simulink model "galvoMdl"  (R2015a)
settings: Solver=ode45  StartTime=0.0  StopTime=10.0  RelTol=1e-3
values from neighbouring files (symbols this model uses):
  JR = 7.3E-9    [dataDict_galvoLSK040EF.sldd]    (also in dataDict_galvoMod6860.sldd = 6.0E-8
  KEL = 0.015    [dataDict_galvoLSK040EF.sldd]    (also in dataDict_galvoMod6860.sldd = 0.0093
  KFR = 4.0E-6    [dataDict_galvoLSK040EF.sldd]    (also in dataDict_galvoMod6860.sldd = 1.0E-10
  L = 0.0018    [dataDict_galvoLSK040EF.sldd]    (also in dataDict_galvoMod6860.sldd = 0.00016
  RL = 2.3    [dataDict_galvoLSK040EF.sldd]    (also in dataDict_galvoMod6860.sldd = 1.5
undefined symbols (not defined in the file or in its folder): KME
settings Model: Creator=mainster  LastModifiedBy=mainster
settings DebuggingCC: UnderspecifiedInitializationDetection=Classic  MergeDetectMultiDrivingBlocksExec=none  SolverPrmCheckMsg=warning  StateNameClashWarn=warning

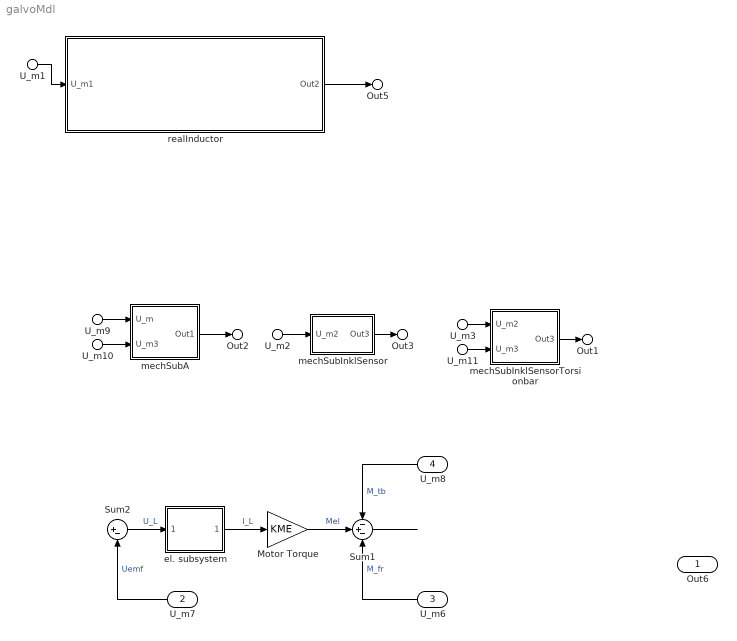
== system galvoMdl ==
  U_m1 : Inport
  U_m7 : Inport  Port=2
  U_m6 : Inport  Port=3
  U_m8 : Inport  Port=4
  U_m9 : Inport  Port=5
  U_m10 : Inport  Port=6
  U_m2 : Inport  Port=7
  U_m3 : Inport  Port=8
  U_m11 : Inport  Port=9
  Motor Torque : Gain  Gain=KME
  Sum1 : Sum  Inputs=-+-
  Sum2 : Sum  Inputs=|+-
  el. subsystem : Subsystem
  mechSubA : Subsystem
  mechSubInklSensor : Subsystem
  mechSubInklSensorTorsionbar : Subsystem
  realInductor : Subsystem
      settings: AttributesFormatString=%<BlockType>
  Out6 : Outport
  Out5 : Outport  Port=2
  Out2 : Outport  Port=3
  Out3 : Outport  Port=4
  Out1 : Outport  Port=5
  wires:
  Sum2/1 -> el. subsystem/1(U_m6)  "U_L"
  U_m7/1 -> Sum2/2  "Uemf"
  ? -> Out6/1
  el. subsystem/1(Out2) -> Motor Torque/1  "I_L"
  Motor Torque/1 -> Sum1/2  "Mel"
  Sum1/1 -> ?
  U_m6/1 -> Sum1/3  "M_fr"
  U_m8/1 -> Sum1/1  "M_tb"
  U_m1/1 -> realInductor/1(U_m1)
  realInductor/1(Out2) -> Out5/1
  U_m9/1 -> mechSubA/1(U_m)
  U_m10/1 -> mechSubA/2(U_m3)
  mechSubA/1(Out1) -> Out2/1
  U_m2/1 -> mechSubInklSensor/1(U_m2)
  mechSubInklSensor/1(Out3) -> Out3/1
  U_m3/1 -> mechSubInklSensorTorsionbar/1(U_m2)
  mechSubInklSensorTorsionbar/1(Out3) -> Out1/1
  U_m11/1 -> mechSubInklSensorTorsionbar/2(U_m3)

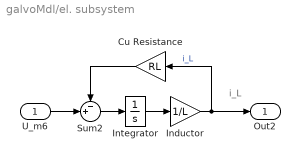
== system galvoMdl/el. subsystem ==
  note: i_L
  U_m6 : Inport
  Cu Resistance : Gain  Gain=RL
  Inductor : Gain  Gain=1/L
  Integrator : Integrator
  Sum2 : Sum  Inputs=-+|
  Out2 : Outport
  wires:
  Inductor/1 -> Cu Resistance/1, Out2/1  "i_L"
  Integrator/1 -> Inductor/1
  Sum2/1 -> Integrator/1
  Cu Resistance/1 -> Sum2/1
  U_m6/1 -> Sum2/2

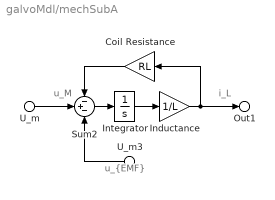
== system galvoMdl/mechSubA ==
  note: u_M
  note: i_L
  note: u_{EMF}
  U_m : Inport
  U_m3 : Inport  Port=2
  Coil Resistance : Gain  Gain=RL
  Inductance : Gain  Gain=1/L
  Integrator : Integrator
  Sum2 : Sum  Inputs=-+-
  Out1 : Outport
  wires:
  Sum2/1 -> Integrator/1
  Coil Resistance/1 -> Sum2/1
  Integrator/1 -> Inductance/1
  U_m3/1 -> Sum2/3
  U_m/1 -> Sum2/2
  Inductance/1 -> Out1/1, Coil Resistance/1

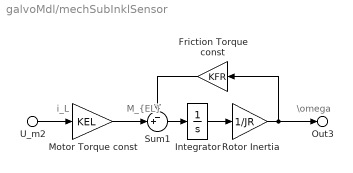
== system galvoMdl/mechSubInklSensor ==
  note: M_{EL}
  note: \omega
  note: i_L
  U_m2 : Inport
  Friction Torque const : Gain  Gain=KFR
  Integrator : Integrator
  Motor Torque const : Gain  Gain=KEL
  Rotor Inertia : Gain  Gain=1/JR
  Sum1 : Sum  Inputs=-+|
  Out3 : Outport
  wires:
  Sum1/1 -> Integrator/1
  Integrator/1 -> Rotor Inertia/1
  Friction Torque const/1 -> Sum1/1
  U_m2/1 -> Motor Torque const/1
  Motor Torque const/1 -> Sum1/2
  Rotor Inertia/1 -> Out3/1, Friction Torque const/1

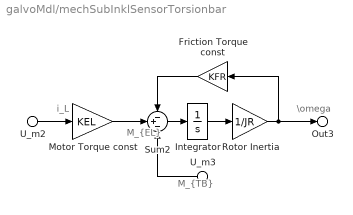
== system galvoMdl/mechSubInklSensorTorsionbar ==
  note: M_{EL}
  note: \omega
  note: i_L
  note: M_{TB}
  U_m2 : Inport
  U_m3 : Inport  Port=2
  Friction Torque const : Gain  Gain=KFR
  Integrator : Integrator
  Motor Torque const : Gain  Gain=KEL
  Rotor Inertia : Gain  Gain=1/JR
  Sum2 : Sum  Inputs=-+-
  Out3 : Outport
  wires:
  Integrator/1 -> Rotor Inertia/1
  Friction Torque const/1 -> Sum2/1
  U_m2/1 -> Motor Torque const/1
  Motor Torque const/1 -> Sum2/2
  Rotor Inertia/1 -> Out3/1, Friction Torque const/1
  U_m3/1 -> Sum2/3
  Sum2/1 -> Integrator/1

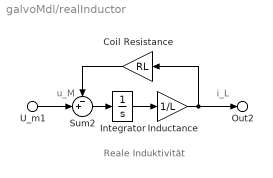
== system galvoMdl/realInductor ==
  note: Reale Induktivität
  note: u_M
  note: i_L
  U_m1 : Inport
  Coil Resistance : Gain  Gain=RL
  Inductance : Gain  Gain=1/L
  Integrator : Integrator
  Sum2 : Sum  Inputs=-+|
  Out2 : Outport
  wires:
  U_m1/1 -> Sum2/2
  Sum2/1 -> Integrator/1
  Inductance/1 -> Out2/1, Coil Resistance/1
  Integrator/1 -> Inductance/1
  Coil Resistance/1 -> Sum2/1
